simulink model "Nr5_sim"  (R2021b)
settings: Solver=VariableStepAuto  StartTime=0.0  StopTime=1  RelTol=1e-3
values from neighbouring files (symbols this model uses):
  A = [0 1;-omegaR^2 -2*xiR*omegaR]    [Nr_5_Mfile.m]
  B = [0;omegaRR^2]    [Nr_5_Mfile.m]
  C = [1 0;0 1;-omegaR^2 -2*xiR*omegaR]    [Nr_5_Mfile.m]
  D = [0; 0;omegaRR^2]    [Nr_5_Mfile.m]
  H = 0.1    [Nr_5_Mfile.m]
undefined symbols (not defined in the file or in its folder): sigbuilder_block
settings Model: Creator=NiBesteh  LastModifiedBy=NiBesteh

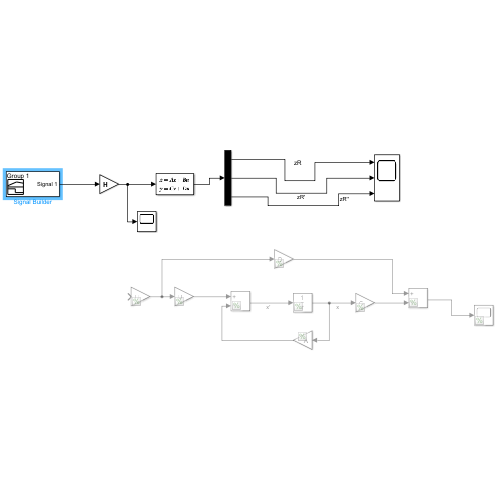
[thumbnail: Simulink's stored preview of the top-level diagram]
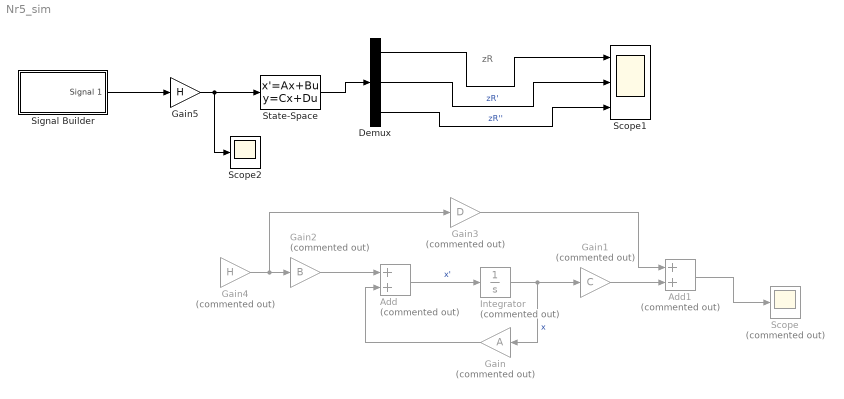
== system Nr5_sim ==
  note: zR
  Add : Sum  Commented=on
  Add1 : Sum  Commented=on
  Demux : Demux  Outputs=3
  Gain : Gain  Commented=on  Gain=A
  Gain1 : Gain  Commented=on  Gain=C
  Gain2 : Gain  Commented=on  Gain=B
  Gain3 : Gain  Commented=on  Gain=D
  Gain4 : Gain  Commented=on  Gain=H
  Gain5 : Gain  Gain=H
  Integrator : Integrator  Commented=on
  Scope : Scope  Commented=on
  Scope1 : Scope  NumInputPorts=3
  Scope2 : Scope
  Signal Builder : Subsystem  Tag=STV Subsys  LoadFcn=sigbuilder_block('load');  StartFcn=sigbuilder_block('start');  StopFcn=sigbuilder_block('stop');  ClipboardFcn=sigbuilder_block('clipboard');  mask(Sigbuilder block){tuvar=[0:10]}
      mask help: Simulink:masks:SigbuilderBlock_MD
      mask init:
      | if ~strcmp(get_param(bdroot(gcbh),'SimulationStatus'),'stopped') tuvar = sigbuilder_block('maskInit'); end
      settings: CopyFcn=sigbuilder_block('copy');  DeleteFcn=sigbuilder_block('delete');  ModelCloseFcn=sigbuilder_block('modelClose');  PreSaveFcn=sigbuilder_block('preSave');  PauseFcn=sigbuilder_block('pause');  ContinueFcn=sigbuilder_block('continue');  NameChangeFcn=sigbuilder_block('namechange');  OpenFcn=sigbuilder_block('open',[437.6 199.2 550.4 400 ]);  CloseFcn=sigbuilder_block('close');
      mask Display: plot(0, 0, 100, 100,[2, 2, 32, 32, 2], [68, 8, 8, 68, 68],[32, 2], [38, 38], [32, 19, 2],[53, 60, 44], [32, 17, 17, 2],[16, 16, 31, 31]);txt = getActiveGroup(gcbh);text(2, 100, txt,'verticalAlignment', 'top');
  State-Space : StateSpace  A=A  B=B  C=C  D=D  InitialCondition=0  AllowTunableDMatrix=on
  wires:
  Add/1 -> Integrator/1  "x'"
  Integrator/1 -> Gain/1, Gain1/1  "x"
  Gain/1 -> Add/2
  Gain1/1 -> Add1/2
  Gain2/1 -> Add/1
  Gain3/1 -> Add1/1
  Gain4/1 -> Gain3/1, Gain2/1
  Add1/1 -> Scope/1
  Signal Builder/1(Signal 1) -> Gain5/1
  Gain5/1 -> Scope2/1, State-Space/1
  State-Space/1 -> Demux/1
  Demux/2 -> Scope1/2  "zR'"
  Demux/3 -> Scope1/3  "zR''"
  Demux/1 -> Scope1/1

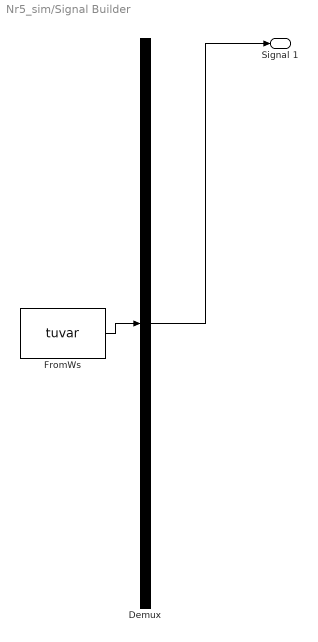
== system Nr5_sim/Signal Builder ==
  Demux : Demux  Tag=STV Demux  Outputs=1
      settings: DisplayOption=none
  FromWs : FromWorkspace  Tag=STV FromWs  VariableName=tuvar
      SigBuilderData=|
      | common.afterFinalStr = 'Extrapolate'
      | common.sampleTime = 0
      | dataSet.timeRange = [0 10]
      | dataSet.name = 'Group 1'
      | sbobj.Groups.Name = 'Group 1'
      | sbobj.Groups.Signals.Name = 'Signal 1'
      | sbobj.Groups.Signals.XData = [0 0.01 0.01 10]
      | sbobj.Groups.Signals.YData = [1 1 0 0]
  Signal 1 : Outport  Tag=STV Outport
  wires:
  Demux/1 -> Signal 1/1
  FromWs/1 -> Demux/1
